simulink model "Safety_filterM_run"  (R2021a)
settings: Solver=ode4  StartTime=0.0  StopTime=15  FixedStep=0.01  RelTol=1e-3
libraries: simulink x1
settings Model: PacingRate=0.500000  Creator=14244039  LastModifiedBy=3054789
settings DebuggingCC: UnderSpecifiedDimensionMsg=warning

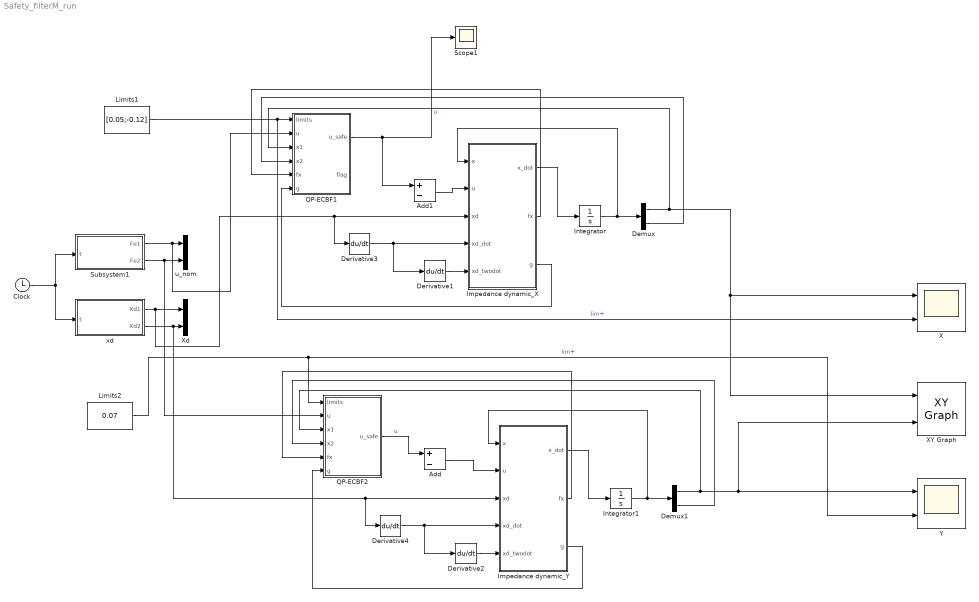
== system Safety_filterM_run ==
  Add : Sum  Inputs=+-
  Add1 : Sum  Inputs=+-
  Clock : Clock
  Demux : Demux  Outputs=2
  Demux1 : Demux  Outputs=2
  Derivative{1..4} (4 alike) : Derivative
  Impedance dynamic_X : MATLAB Function  TreatAsAtomicUnit=on
  Impedance dynamic_Y : MATLAB Function  TreatAsAtomicUnit=on
  Integrator : Integrator  InitialCondition=[0.0;0]
  Integrator1 : Integrator  InitialCondition=[0.16;0]
  Limits1 : Constant  Value=[0.05;-0.12]  VectorParams1D=off  SampleTime=-1
  Limits2 : Constant  Value=0.07  VectorParams1D=off  SampleTime=-1
  QP-ECBF1 : Subsystem
  QP-ECBF2 : Subsystem
  Scope1 : Scope
  Subsystem1 : Subsystem
  X : Scope  NumInputPorts=2
  XY Graph : simulink/Sinks/XY Graph  xmin=-1  xmax=1  ymin=-1  ymax=1  st=-1
  Xd : Mux  Inputs=2
  Y : Scope  NumInputPorts=2
  u_nom : Mux  Inputs=2
  xd : MATLAB Function  TreatAsAtomicUnit=on
  wires:
  xd/1(Xd1) -> Impedance dynamic_X/3(xd), Derivative3/1, Xd/1
  Subsystem1/1(Fe1) -> QP-ECBF1/2(u), u_nom/1
  Clock/1 -> xd/1(t), Subsystem1/1(t)
  Derivative3/1 -> Impedance dynamic_X/4(xd_dot), Derivative1/1
  Derivative1/1 -> Impedance dynamic_X/5(xd_twodot)
  Impedance dynamic_X/1(x_dot) -> Integrator/1
  Integrator/1 -> Demux/1, Impedance dynamic_X/1(x)
  Demux/1 -> QP-ECBF1/3(x1), XY Graph/1, X/1
  Limits1/1 -> X/2, QP-ECBF1/1(limits)  "lim+"
  Demux/2 -> QP-ECBF1/4(x2)
  QP-ECBF1/1(u_safe) -> Add1/1, Scope1/1  "u"
  Impedance dynamic_X/2(fx) -> QP-ECBF1/5(fx)
  Impedance dynamic_X/3(g) -> QP-ECBF1/6(g)
  Impedance dynamic_Y/3(g) -> QP-ECBF2/6(g)
  Impedance dynamic_Y/2(fx) -> QP-ECBF2/5(fx)
  QP-ECBF2/1(u_safe) -> Add/1  "u"
  Demux1/2 -> QP-ECBF2/4(x2)
  Demux1/1 -> QP-ECBF2/3(x1), XY Graph/2, Y/1
  xd/2(Xd2) -> Impedance dynamic_Y/3(xd), Derivative4/1, Xd/2
  Limits2/1 -> QP-ECBF2/1(limits), Y/2  "lim+"
  Impedance dynamic_Y/1(x_dot) -> Integrator1/1
  Derivative4/1 -> Impedance dynamic_Y/4(xd_dot), Derivative2/1
  Derivative2/1 -> Impedance dynamic_Y/5(xd_twodot)
  Integrator1/1 -> Demux1/1, Impedance dynamic_Y/1(x)
  Subsystem1/2(Fe2) -> QP-ECBF2/2(u), u_nom/2
  Add/1 -> Impedance dynamic_Y/2(u)
  Add1/1 -> Impedance dynamic_X/2(u)

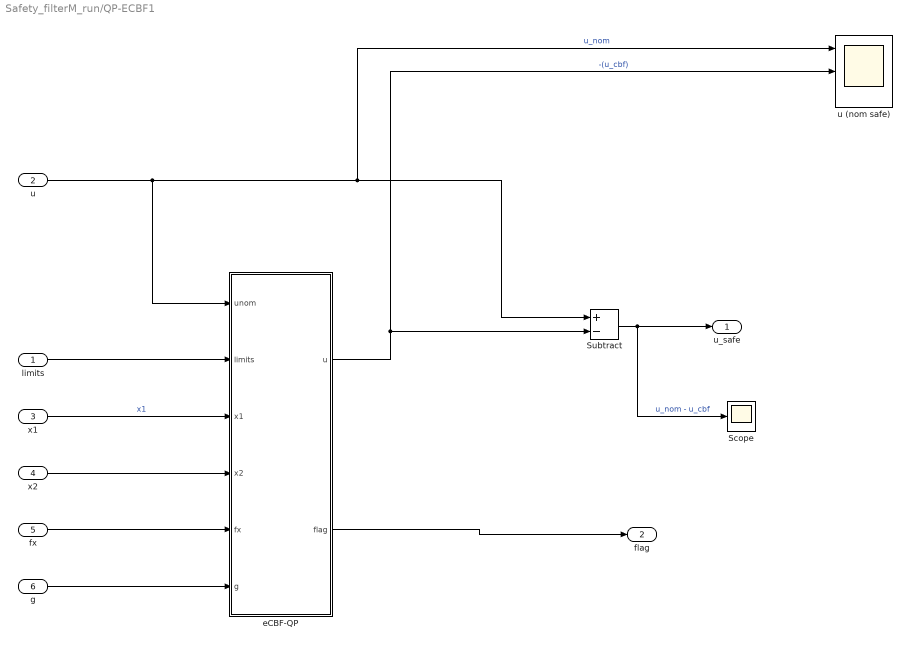
== system Safety_filterM_run/QP-ECBF1 ==
  limits : Inport
  u : Inport  Port=2
  x1 : Inport  Port=3
  x2 : Inport  Port=4
  fx : Inport  Port=5
  g : Inport  Port=6
  Scope : Scope
  Subtract : Sum  Inputs=+-
  eCBF-QP : MATLAB Function  TreatAsAtomicUnit=on
  u (nom safe) : Scope  NumInputPorts=3
  u_safe : Outport
  flag : Outport  Port=2
  wires:
  x2/1 -> eCBF-QP/4(x2)
  limits/1 -> eCBF-QP/2(limits)
  u/1 -> eCBF-QP/1(unom), Subtract/1, u (nom safe)/1  "u_nom"
  x1/1 -> eCBF-QP/3(x1)  "x1"
  eCBF-QP/1(u) -> Subtract/2, u (nom safe)/2  "-(u_cbf)"
  Subtract/1 -> u_safe/1, Scope/1  "u_nom - u_cbf"
  fx/1 -> eCBF-QP/5(fx)
  g/1 -> eCBF-QP/6(g)
  eCBF-QP/2(flag) -> flag/1

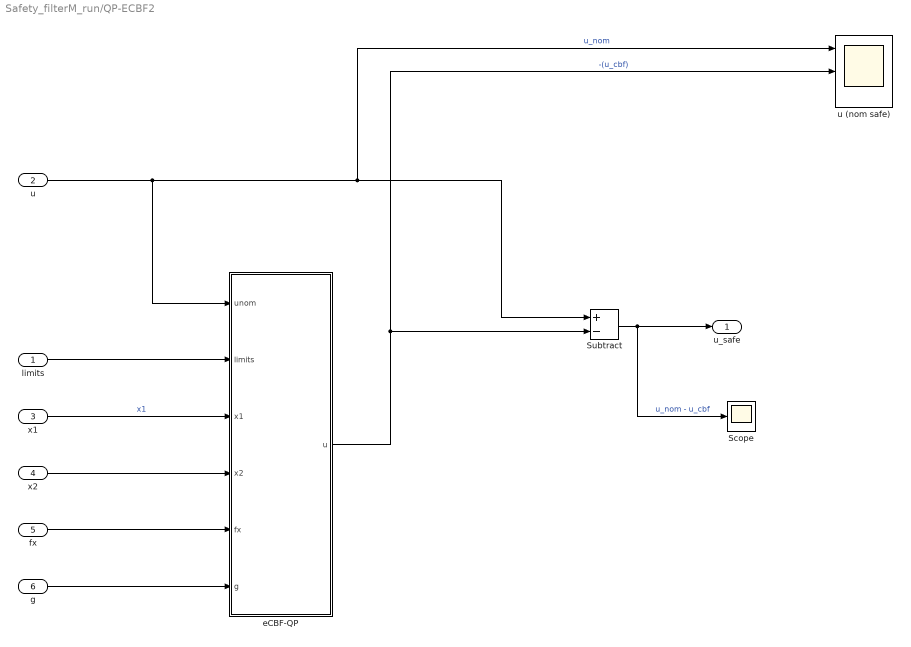
== system Safety_filterM_run/QP-ECBF2 ==
  limits : Inport
  u : Inport  Port=2
  x1 : Inport  Port=3
  x2 : Inport  Port=4
  fx : Inport  Port=5
  g : Inport  Port=6
  Scope : Scope
  Subtract : Sum  Inputs=+-
  eCBF-QP : MATLAB Function  TreatAsAtomicUnit=on
  u (nom safe) : Scope  NumInputPorts=3
  u_safe : Outport
  wires:
  x2/1 -> eCBF-QP/4(x2)
  limits/1 -> eCBF-QP/2(limits)
  u/1 -> eCBF-QP/1(unom), Subtract/1, u (nom safe)/1  "u_nom"
  x1/1 -> eCBF-QP/3(x1)  "x1"
  eCBF-QP/1(u) -> Subtract/2, u (nom safe)/2  "-(u_cbf)"
  Subtract/1 -> u_safe/1, Scope/1  "u_nom - u_cbf"
  fx/1 -> eCBF-QP/5(fx)
  g/1 -> eCBF-QP/6(g)

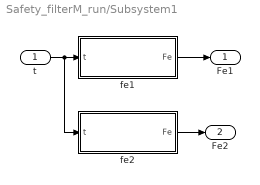
== system Safety_filterM_run/Subsystem1 ==
  t : Inport
  fe1 : MATLAB Function  TreatAsAtomicUnit=on
  fe2 : MATLAB Function  TreatAsAtomicUnit=on
  Fe1 : Outport
  Fe2 : Outport  Port=2
  wires:
  fe1/1(Fe) -> Fe1/1
  fe2/1(Fe) -> Fe2/1
  t/1 -> fe2/1(t), fe1/1(t)

== matlab function Safety_filterM_run/Impedance dynamic_Y ==
  data: x input size=[2 1]; u input; x_dot output size=[2 1]; xd input; xd_dot input; xd_twodot input; fx output; g output
function [x_dot,fx,g] = System(x,u,xd,xd_dot,xd_twodot)

    km = 20;
    kb = 20;                                                       
    kk = 100;
    fx = [x(2);
        -(1/km)*(kb*(x(2)-xd_dot)+kk*(x(1)-xd)-km*xd_twodot)];
    g = [0;km^(-1)];
    x_dot = fx + g*u;
end

== matlab function Safety_filterM_run/Subsystem1/fe1 ==
  data: t input; Fe output
function Fe  = External_force(t)

   Fe = 0*(t<4|t>=11) + (1-cos(pi*t))*(t>=4&t<5) + 2*(t>=5&t<10) + (1+cos(pi*t))*(t>=10&t<11);

end

== matlab function Safety_filterM_run/QP-ECBF2/eCBF-QP ==
  settings: updateMethod=DISCRETE
  data: unom input; limits input; u output size=1; x1 input; x2 input; fx input; g input
function u = fcn(unom, limits, x1, x2,fx,g)
     %Barrier Limits
    lim     = limits(1);
 
    %ECBF Gains
    k1      = 20;
    k2      = 100;
    
    % Maximum Value CBF variables
    hx      = (x1 - lim)^2 - 0.001 ;  %(lim^2 - x1^2) 
    Lfhx    = 2*(x1 - lim)*x2;
    
%     L2fhx   = 2*(x1 - lim)*((2*x1*(x1^2 + x2)) + x1*x2 + x1 + (1 + x1^2)*CTL) + 2*(x1^2 + x2)^2;
%     eCBF    = L2fhx + k1*Lfhx + k2*hx;
    
    
    H       = [2];
    f       = [0]; 
    
    A       = [2*(x1-lim)*g(2)]; 
            
    b       = [ 2*(x1 - lim) * ( fx(2)+ g(2)*unom) + 2*x2 + k1*Lfhx + k2*hx];
    
    X   = 0;
    flag = 0;
    coder.extrinsic('quadprog');
    [output, ~, flag]   = quadprog(H,f,A,b,[],[],[],[]);

    if flag == 1
        X = output;
    else
        X   = 0;
    end
    
%Function outputs
    u = X(1); 
end

== matlab function Safety_filterM_run/Subsystem1/fe2 ==
  data: t input; Fe output
function Fe  = External_force(t)

   Fe = 0*(t<4|t>=11) + 2*(1-cos(pi*t))*(t>=4&t<5) + 4*(t>=5&t<10) + 2*(1+cos(pi*t))*(t>=10&t<11);

end

== matlab function Safety_filterM_run/xd ==
  data: t input; Xd1 output; Xd2 output
function [Xd1, Xd2] = Desired_traj(t)

    Xd1=0.14*cos(0.5*t);
    Xd2=0.14*sin(0.5*t);
    
end

== matlab function Safety_filterM_run/QP-ECBF1/eCBF-QP ==
  settings: updateMethod=DISCRETE
  data: unom input; limits input; u output size=1; x1 input; x2 input; fx input; g input; flag output
function [u,flag] = fcn(unom, limits, x1, x2,fx,g)
     %Barrier Limits
    lim     = limits(1);
    lim2    = limits(2);
 
    %ECBF Gains
    k1      = 50;
    k2      = 300;
    
    k3      = 50;
    k4      = 300;
    % Maximum Value CBF variables
    hx      = (x1 - lim)^2 - 0.001 ;  %(lim^2 - x1^2) 
    Lfhx    = 2*(x1 - lim)*x2;
    
%     L2fhx   = 2*(x1 - lim)*((2*x1*(x1^2 + x2)) + x1*x2 + x1 + (1 + x1^2)*CTL) + 2*(x1^2 + x2)^2;
%     eCBF    = L2fhx + k1*Lfhx + k2*hx;
    
    % Minimum Value CBF variables
    hx2     = (lim2 - x1)^2 - 0.001 ;  %(lim^2 - x1^2) 
    Lfhx2    = -2*(lim2 - x1)*x2;


    H       = [2 0; 0 0];
    f       = [0;0]; 
    
    A       = [2*(x1-lim)*g(2) 0;
              -2*(lim2 - x1)*g(2) 0]; 
            
    b       = [ 2*(x1 - lim) * ( fx(2)+ g(2)*unom) + 2*x2 + k1*Lfhx + k2*hx;
               -2*(lim2 - x1) * ( fx(2)+ g(2)*unom) + 2*x2 + k3*Lfhx2 + k4*hx2];
    X   = [0;0];
    flag = 0;
    coder.extrinsic('quadprog');
    [output, ~, flag]   = quadprog(H,f,A,b,[],[],[],[]);

    if flag == 1
        X = output;
    else
        X   = [0;0];
    end
    
%Function outputs
    u = X(1); 
end

== matlab function Safety_filterM_run/Impedance dynamic_X ==
  data: x input size=[2 1]; u input; x_dot output size=[2 1]; xd input; xd_dot input; xd_twodot input; fx output; g output
function [x_dot,fx,g] = System(x,u,xd,xd_dot,xd_twodot)

    km = 20;
    kb = 20;                                                       
    kk = 100;
    fx = [x(2);
        -(1/km)*(kb*(x(2)-xd_dot)+kk*(x(1)-xd)-km*xd_twodot)];
    g = [0;km^(-1)];
    x_dot = fx + g*u;
end
